simulink model "ActuatorControlSystem"  (R2022a)
settings: Solver=VariableStepAuto  StartTime=0.0  StopTime=10.0  RelTol=1e-3
undefined symbols (not defined in the file or in its folder): A, B, C, D
libraries: simulink x2, slpidlib x1, discretizing x1
settings Model: Creator=ebert  LastModifiedBy=ebert

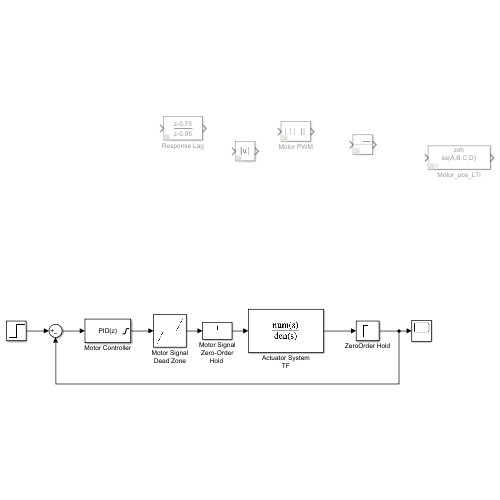
[thumbnail: Simulink's stored preview of the top-level diagram]
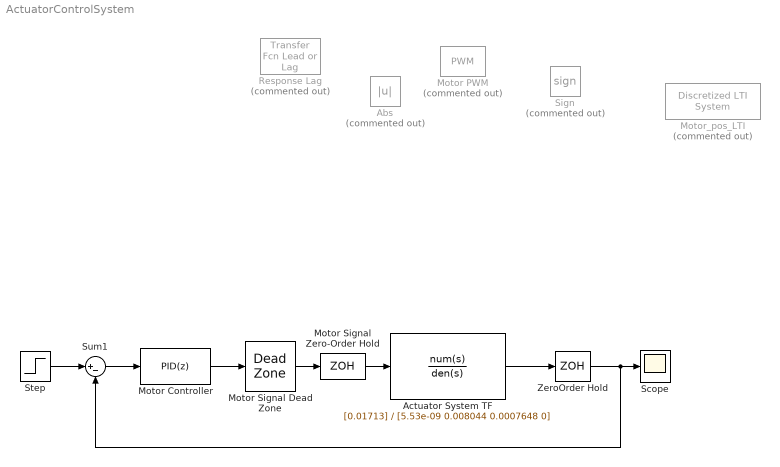
== system ActuatorControlSystem ==
  Abs : Abs  Commented=on  SaturateOnIntegerOverflow=off
  Actuator System TF : TransferFcn  Numerator=[0.01713]  Denominator=[5.53e-09 0.008044 0.0007648 0]
  Motor Controller : slpidlib/PID Controller  Controller=PID  Form=Parallel  TimeDomain=Discrete-time  UseExternalTs=off  SampleTime=1/30  IntegratorMethod=Forward Euler  FilterMethod=Forward Euler  ControllerParametersSource=internal  P=11.601730053616  I=1.65851993442092  UseKiTs=off  D=8.32594106652751  N=37.6592705634507  UseFilter=on  TunerSelectOption=Transfer Function Based (PID Tuner App)  InitialConditionSource=internal  InitialConditionForIntegrator=0  InitialConditionForFilter=0  DifferentiatorICPrevScaledInput=0  ExternalReset=none  TrackingMode=off  Kt=1  LimitOutput=on  SatLimitsSource=internal  UpperSaturationLimit=0.9  LowerSaturationLimit=-0.9  LinearizeAsGain=off  AntiWindupMode=clamping  Kb=1  POutMin=[]  POutMax=[]  IOutMin=[]  IOutMax=[]  DOutMin=[]  DOutMax=[]  NOutMin=[]  NOutMax=[]  SumOutMin=[]  SumOutMax=[]  SaturationOutMin=[]  SaturationOutMax=[]  PParamMin=[]  PParamMax=[]  IParamMin=[]  IParamMax=[]  DParamMin=[]  DParamMax=[]  NParamMin=[]  NParamMax=[]  KbParamMin=[]  KbParamMax=[]  KtParamMin=[]  KtParamMax=[]  KbOutMin=[]  KbOutMax=[]  KtOutMin=[]  KtOutMax=[]  IntegratorOutMin=[]  IntegratorOutMax=[]  FilterOutMin=[]  FilterOutMax=[]  SumI1OutMin=[]  SumI1OutMax=[]  SumI2OutMin=[]  SumI2OutMax=[]  SumI3OutMin=[]  SumI3OutMax=[]  SumI4OutMin=[]  SumI4OutMax=[]  SumDOutMin=[]  SumDOutMax=[]  DifferentiatorOutMin=[]  DifferentiatorOutMax=[]  FilterDiffOutCoefMin=[]  FilterDiffOutCoefMax=[]  ReciprocalOutMin=[]  ReciprocalOutMax=[]  SumDenOutMin=[]  SumDenOutMax=[]  SumNumOutMin=[]  SumNumOutMax=[]  DivideOutMin=[]  DivideOutMax=[]  UdiffTsProdOutMin=[]  UdiffTsProdOutMax=[]  NTsProdOutMin=[]  NTsProdOutMax=[]  UintegralTsProdOutMin=[]  UintegralTsProdOutMax=[]  UngainTsProdOutMin=[]  UngainTsProdOutMax=[]  IntegratorContinuousStateAttributes=''  IntegratorStateMustResolveToSignalObject=off  IntegratorRTWStateStorageClass=Auto  FilterContinuousStateAttributes=''  FilterStateMustResolveToSignalObject=off  FilterRTWStateStorageClass=Auto  ParallelPVariant=InternalParameters  IdealPVariant=Disabled  IVariant=InternalParameters  DVariant=InternalParameters  IntegratorVariant=Discrete  SatVariant=Enabled  AWVariant=DiscClampingParallel  PCopyVariant=Disabled  TRVariant=Disabled  FdbkBlocksVariant=Forward  IdealPFdbkVariant=Disabled  SatFdbkVariant=Disabled  DerivativeFilterVariant=ForwardEulerFilter  NVariant=InternalParameters  NCopyVariant=Disabled  FilterICVariant=InternalICsFilter  IntegratorICVariant=InternalICs  ExternalResetVariant=Disabled  TRSumVariant=Passthrough  SumFdbkVariant=Disabled  SumVariant=Sum_PID  TsampFilterVariant=InternalTs  TsampNgainVariant=Passthrough  TsampIntegralVariant=Passthrough  ExternalSaturationOutDataTypeStr=Inherit: Same as second input  aMode=0
  Motor PWM : simulink/Discontinuities/PWM  Commented=on  DisableCoverage=on  Period=1  DisallowZeroDutyCycle=off  RunAtFixedTimeIntervals=off  SampleTime=0.1
  Motor Signal Dead Zone : DeadZone  LowerValue=-0.1  UpperValue=0.1
  "Motor Signal Zero-Order Hold " : ZeroOrderHold  SampleTime=-1
  Motor_pos_LTI : discretizing/Discretized LTI System  Commented=on  sysc=ss(A,B,C,D)  cic=[0]  SampleTime=1/30  method=zoh  Wc=0
      settings: SourceProductBaseCode=SL
  Response Lag : simulink/Discrete/Transfer Fcn Lead or Lag  Commented=on  PoleZ=0.95  ZeroZ=0.75  ICPrevOutput=0.0  ICPrevInput=0.0  DoSatur=off
      settings: SourceProductBaseCode=SL
  Scope : Scope
  Sign : Signum  Commented=on
  Step : Step
  Sum1 : Sum  Inputs=|+-
  ZeroOrder Hold : ZeroOrderHold  SampleTime=-1
  wires:
  Motor Signal Dead Zone/1 -> "Motor Signal Zero-Order Hold "/1
  Step/1 -> Sum1/1
  ZeroOrder Hold/1 -> Sum1/2, Scope/1
  "Motor Signal Zero-Order Hold "/1 -> Actuator System TF/1
  Actuator System TF/1 -> ZeroOrder Hold/1
  Sum1/1 -> Motor Controller/1
  Motor Controller/1 -> Motor Signal Dead Zone/1
